simulink model "P1_simspaceship_eulr_v2"  (Simulink 7.8)
settings: Solver=ode45  StartTime=0  StopTime=tf  FixedStep=dt_sim  RelTol=1e-6
undefined symbols (not defined in the file): JB, K, X0
libraries: vrlib x1
settings Model: Creator=vickTJ  LastModifiedBy=Dan  BufferReuse=off
settings SolverCC: MaxConsecutiveMinStep=3
settings DataIOCC: ExternalInput=a  InitialState=[]  LimitDataPoints=off  MaxDataPoints=5000  SaveState=on  SignalLogging=off  DSMLogging=off  StateSaveName=stout
settings OptimizationCC: InlineParams=on  BufferReuse=off
settings DebuggingCC: SolverPrmCheckMsg=none  FcnCallInpInsideContextMsg=Use local settings  UnconnectedInputMsg=none  UnconnectedOutputMsg=none  InitInArrayFormatMsg=none  SFInvalidInputDataAccessInChartInitDiag=none

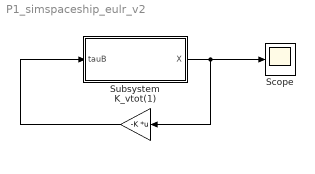
== system P1_simspaceship_eulr_v2 ==
  K_vtot(1) : Gain  Gain=-K  Multiplication=Matrix(K*u)
  Scope : Scope
  Subsystem : Subsystem
  wires:
  K_vtot(1)/1 -> Subsystem/1(tauB)
  Subsystem/1(X) -> K_vtot(1)/1, Scope/1

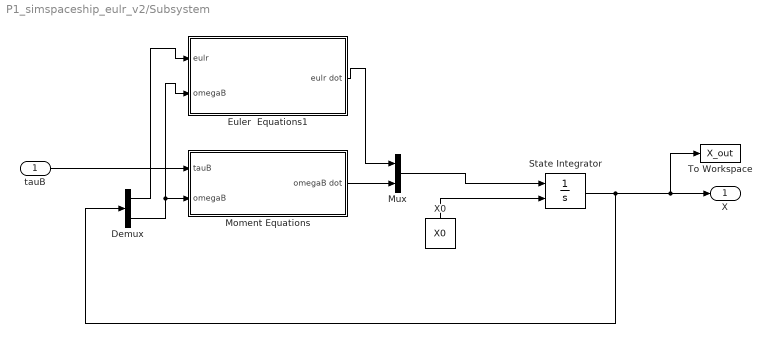
== system P1_simspaceship_eulr_v2/Subsystem ==
  tauB : Inport
  Demux : Demux  Outputs=2
  Euler  Equations1 : Subsystem
  Moment Equations : Subsystem
  Mux : Mux  Inputs=2
  State Integrator : Integrator  InitialConditionSource=external
  To Workspace : ToWorkspace  VariableName=X_out  SampleTime=-1  SaveFormat=Structure
  X0 : Constant  Value=X0
  X : Outport
  wires:
  X0/1 -> State Integrator/2
  State Integrator/1 -> Demux/1, X/1, To Workspace/1
  Demux/1 -> Euler  Equations1/1(eulr)
  Demux/2 -> Moment Equations/2(omegaB), Euler  Equations1/2(omegaB)
  Euler  Equations1/1(eulr dot) -> Mux/1
  Moment Equations/1(omegaB dot) -> Mux/2
  Mux/1 -> State Integrator/1
  tauB/1 -> Moment Equations/1(tauB)

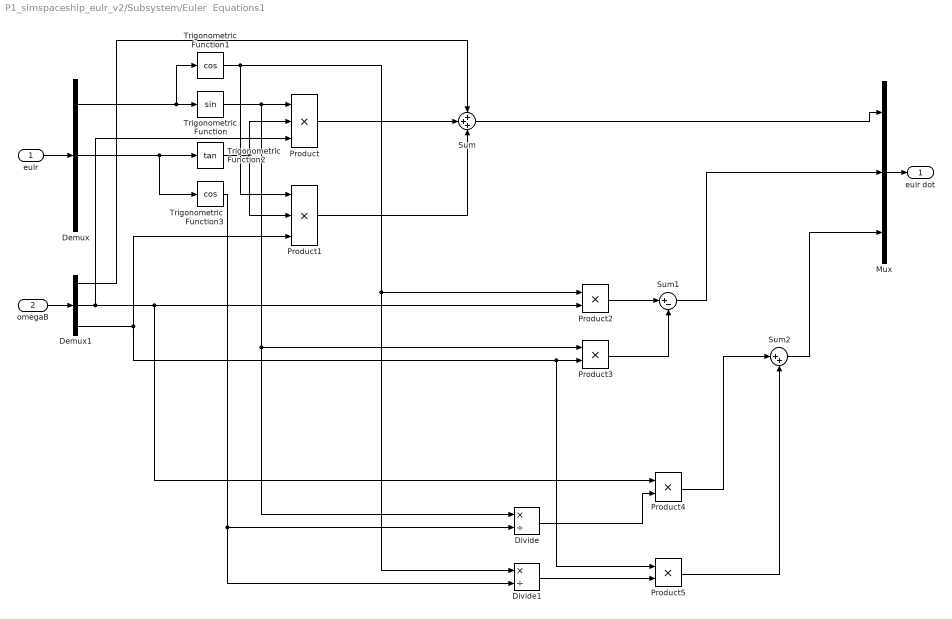
== system P1_simspaceship_eulr_v2/Subsystem/Euler  Equations1 ==
  eulr : Inport
  omegaB : Inport  Port=2
  Demux : Demux  Outputs=3
  Demux1 : Demux  Outputs=3
  Divide : Product  Inputs=*/
  Divide1 : Product  Inputs=*/
  Mux : Mux  Inputs=3
  Product : Product  Inputs=3  RndMeth=Zero
  Product1 : Product  Inputs=3  RndMeth=Zero
  Product{2..5} (4 alike) : Product  RndMeth=Zero
  Sum : Sum  Inputs=+++
  Sum1 : Sum  Inputs=|+-
  Sum2 : Sum  Inputs=|++
  Trigonometric Function : Trigonometry
  Trigonometric Function1 : Trigonometry  Operator=cos
  Trigonometric Function2 : Trigonometry  Operator=tan
  Trigonometric Function3 : Trigonometry  Operator=cos
  eulr dot : Outport
  wires:
  eulr/1 -> Demux/1
  omegaB/1 -> Demux1/1
  Mux/1 -> eulr dot/1
  Demux/2 -> Trigonometric Function2/1, Trigonometric Function3/1
  Demux/1 -> Trigonometric Function1/1, Trigonometric Function/1
  Trigonometric Function/1 -> Product/1, Product3/1, Divide/1
  Trigonometric Function2/1 -> Product/2, Product1/2
  Demux1/2 -> Product/3, Product2/2, Product4/1
  Sum/1 -> Mux/1
  Product1/1 -> Sum/3
  Trigonometric Function1/1 -> Divide1/1, Product2/1, Product1/1
  Demux1/3 -> Product1/3, Product3/2, Product5/1
  Product2/1 -> Sum1/1
  Product3/1 -> Sum1/2
  Sum1/1 -> Mux/2
  Trigonometric Function3/1 -> Divide/2, Divide1/2
  Divide/1 -> Product4/2
  Product4/1 -> Sum2/1
  Sum2/1 -> Mux/3
  Demux1/1 -> Sum/1
  Product/1 -> Sum/2
  Divide1/1 -> Product5/2
  Product5/1 -> Sum2/2

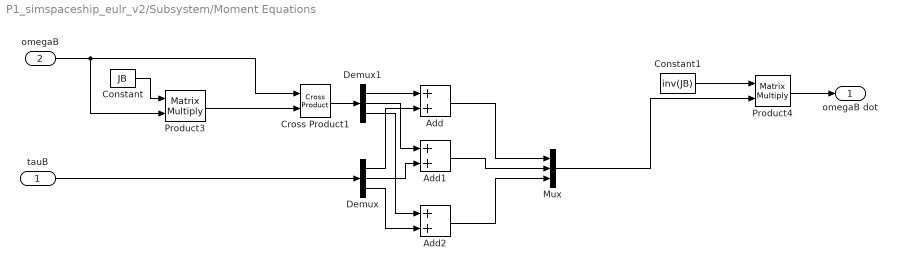
== system P1_simspaceship_eulr_v2/Subsystem/Moment Equations ==
  tauB : Inport  OutDataTypeStr=double
  omegaB : Inport  Port=2
  Add : Sum
  Add1 : Sum
  Add2 : Sum
  Constant : Constant  Value=JB
  Constant1 : Constant  Value=inv(JB)
  Cross Product1 : vrlib/Utilities/Cross Product
  Demux : Demux  Outputs=3
  Demux1 : Demux  Outputs=3
  Mux : Mux  Inputs=3
  Product3 : Product  Multiplication=Matrix(*)  RndMeth=Zero
  Product4 : Product  Multiplication=Matrix(*)  RndMeth=Zero
  omegaB dot : Outport
  wires:
  Product4/1 -> omegaB dot/1
  Constant/1 -> Product3/1
  omegaB/1 -> Product3/2, Cross Product1/1
  Product3/1 -> Cross Product1/2
  Constant1/1 -> Product4/1
  tauB/1 -> Demux/1
  Cross Product1/1 -> Demux1/1
  Demux1/1 -> Add/1
  Demux/1 -> Add/2
  Demux1/2 -> Add1/1
  Demux/2 -> Add1/2
  Demux1/3 -> Add2/1
  Demux/3 -> Add2/2
  Add/1 -> Mux/1
  Add1/1 -> Mux/2
  Add2/1 -> Mux/3
  Mux/1 -> Product4/2
